simulink model "claseAutoPIDzigler"  (R2018a)
settings: Solver=VariableStepAuto  StartTime=0.0  StopTime=tfn  MaxStep=0.001  RelTol=1e-3
values from neighbouring files (symbols this model uses):
  A = 1    [Control.m]
  den = [tao 1]    [Control.m]
  Kc1 = (0.902/kp)*((th/tao)^-0.985)    (= 3.10237884114)    [Control.m]
  Kc2 = ((0.984/kp)*((th/tao)^-0.986))*0.1    (= 0.339058027753)    [Control.m]
  Kc3 = ((1.435/kp)*((th/tao)^-0.921))*0.1    (= 0.439277724982)    [Control.m]
  num = kp    (= 1.747)    [Control.m]
  Td3 = (0.482*tao)*((th/tao)^1.137)    (= 1.71650648061)    [Control.m]
  th = 4.57    [Control.m]
  Ti2 = (tao/0.608)*((th/tao)^0.707)    (= 12.8135768499)    [Control.m]
  Ti3 = (tao/0.878)*((th/tao)^0.749)    (= 8.22001343401)    [Control.m]
  Tup = 1    [Control.m]
libraries: simulink x1
settings Model: Creator=b3s217e5  LastModifiedBy=b3s217e5
settings DebuggingCC: LibraryContextMissingDiagnostic=warning
settings SFSimCC: SimUseLocalCustomCode=on
settings RTWCC: RTWUseLocalCustomCode=on

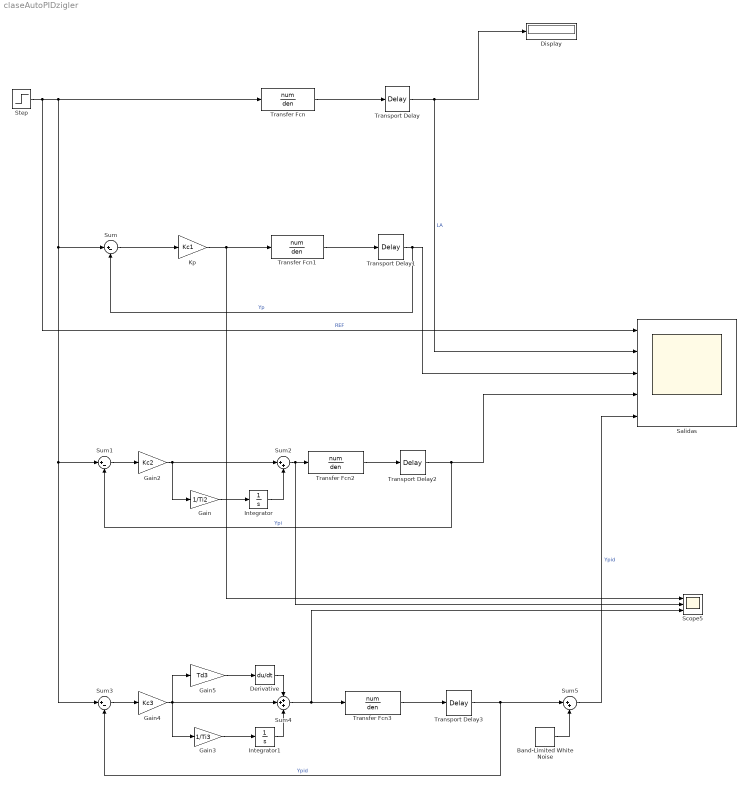
== system claseAutoPIDzigler ==
  Band-Limited White Noise : simulink/Sources/Band-Limited White Noise  Cov=pruido  Ts=0.1  seed=[23341]
  Derivative : Derivative
  Display : Display
      settings: Decimation=2
  Gain : Gain  Gain=1/Ti2
  Gain2 : Gain  Gain=Kc2
  Gain3 : Gain  Gain=1/Ti3
  Gain4 : Gain  Gain=Kc3
  Gain5 : Gain  Gain=Td3
  Integrator : Integrator
  Integrator1 : Integrator
  Kp : Gain  Gain=Kc1
  Salidas : Scope  NumInputPorts=5
  Scope5 : Scope  NumInputPorts=3
  Step : Step  Time=Tup  After=A  SampleTime=0
  Sum : Sum  Inputs=|+-
  Sum1 : Sum  Inputs=|+-
  Sum2 : Sum  Inputs=|++
  Sum3 : Sum  Inputs=|+-
  Sum4 : Sum  Inputs=+++
  Sum5 : Sum  Inputs=|++
  Transfer Fcn{,1..3} (4 alike) : TransferFcn  Numerator=num  Denominator=den
  Transport Delay{,1..3} (4 alike) : TransportDelay  DelayTime=th
  wires:
  Transfer Fcn/1 -> Transport Delay/1
  Transport Delay/1 -> Salidas/2, Display/1  "LA"
  Transfer Fcn1/1 -> Transport Delay1/1
  Transport Delay1/1 -> Salidas/3, Sum/2  "Yp"
  Sum/1 -> Kp/1
  Sum1/1 -> Gain2/1
  Transfer Fcn2/1 -> Transport Delay2/1
  Transport Delay2/1 -> Sum1/2, Salidas/4  "Ypi"
  Gain/1 -> Integrator/1
  Sum2/1 -> Scope5/2, Transfer Fcn2/1
  Gain2/1 -> Gain/1, Sum2/1
  Integrator/1 -> Sum2/2
  Gain4/1 -> Gain3/1, Sum4/2, Gain5/1
  Gain3/1 -> Integrator1/1
  Transfer Fcn3/1 -> Transport Delay3/1
  Step/1 -> Salidas/1, Transfer Fcn/1, Sum1/1, Sum3/1, Sum/1  "REF"
  Transport Delay3/1 -> Sum5/1, Sum3/2  "Ypid"
  Sum3/1 -> Gain4/1
  Integrator1/1 -> Sum4/3
  Gain5/1 -> Derivative/1
  Derivative/1 -> Sum4/1
  Band-Limited White Noise/1 -> Sum5/2
  Sum5/1 -> Salidas/5  "Ypid"
  Kp/1 -> Scope5/1, Transfer Fcn1/1
  Sum4/1 -> Scope5/3, Transfer Fcn3/1
